simulink model "PropuestaControl"  (R2022b)
settings: Solver=ode4  StartTime=0.0  StopTime=60  FixedStep=0.001  RelTol=1e-3
values from neighbouring files (symbols this model uses):
  Ap = Am(:,1:20)    [IniciadorParametros.m]
  B = [zeros(n,n);eye(n,n)]    [IniciadorParametros.m]
  Psi1 = [V1 zeros(n,n)]    [IniciadorParametros.m]
  Psi2 = [zeros(n,n) V2]    [IniciadorParametros.m]
  V0 = Data(:,1)    [IniciadorParametros.m]
undefined symbols (not defined in the file or in its folder): A, P, W1, W2
settings Model: Creator=raul  LastModifiedBy=raul

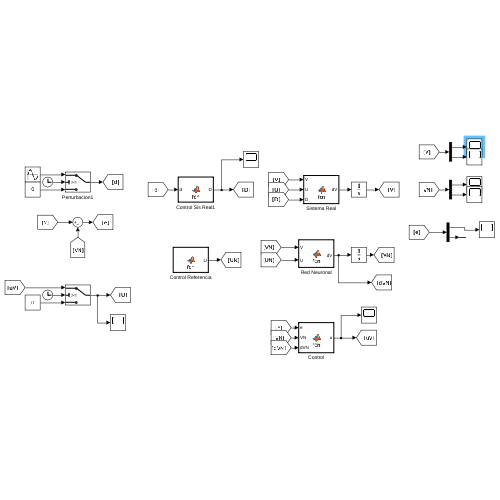
[thumbnail: Simulink's stored preview of the top-level diagram]
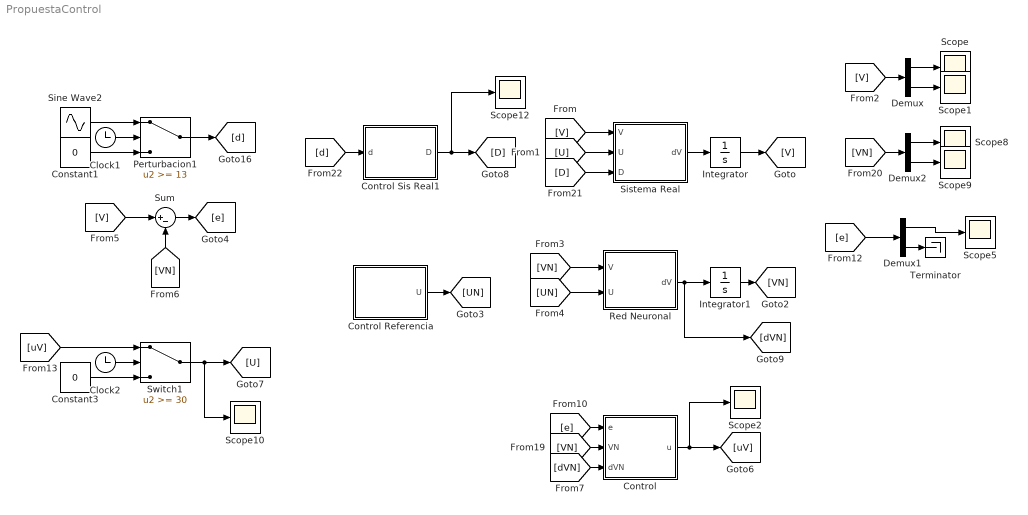
== system PropuestaControl ==
  Clock1 : Clock
  Clock2 : Clock
  Constant1 : Constant  Value=0
  Constant3 : Constant  Value=0
  Control : MATLAB Function  TreatAsAtomicUnit=on
  Control Referencia : MATLAB Function  TreatAsAtomicUnit=on
  Control Sis Real1 : MATLAB Function  TreatAsAtomicUnit=on
  Demux : Demux  Outputs=2
  Demux1 : Demux  Outputs=2
  Demux2 : Demux  Outputs=2
  Integrator : Integrator  InitialCondition=V0
  Integrator1 : Integrator  InitialCondition=V0
  Perturbacion1 : Switch  Threshold=13  SaturateOnIntegerOverflow=off  InputSameDT=off
  Red Neuronal : MATLAB Function  TreatAsAtomicUnit=on
  Scope{,1..2,5,8..10,12} (8 alike) : Scope
  Sine Wave2 : Sin  Frequency=5  SampleTime=0
  Sistema Real : MATLAB Function  TreatAsAtomicUnit=on
  Sum : Sum  Inputs=|+-
  Switch1 : Switch  Threshold=30  SaturateOnIntegerOverflow=off  InputSameDT=off
  Terminator : Terminator
  wires:
  Sistema Real/1(dV) -> Integrator/1
  Integrator/1 -> [V]
  [V] -> Sistema Real/1(V)
  [U] -> Sistema Real/2(U)
  [V] -> Demux/1
  Demux/1 -> Scope/1
  Demux/2 -> Scope1/1
  [VN] -> Red Neuronal/1(V)
  Red Neuronal/1(dV) -> [dVN], Integrator1/1
  Integrator1/1 -> [VN]
  [V] -> Sum/1
  [VN] -> Sum/2
  Perturbacion1/1 -> [d]
  Sine Wave2/1 -> Perturbacion1/1
  Clock1/1 -> Perturbacion1/2
  Constant1/1 -> Perturbacion1/3
  [UN] -> Red Neuronal/2(U)
  Control Referencia/1(U) -> [UN]
  Sum/1 -> [e]
  [e] -> Control/1(e)
  Control/1(u) -> Scope2/1, [uV]
  Switch1/1 -> Scope10/1, [U]
  Constant3/1 -> Switch1/3
  Clock2/1 -> Switch1/2
  [e] -> Demux1/1
  Demux1/1 -> Scope5/1
  Demux1/2 -> Terminator/1
  [VN] -> Control/2(VN)
  Demux2/1 -> Scope8/1
  Demux2/2 -> Scope9/1
  [VN] -> Demux2/1
  [uV] -> Switch1/1
  Control Sis Real1/1(D) -> Scope12/1, [D]
  [d] -> Control Sis Real1/1(d)
  [D] -> Sistema Real/3(D)
  [dVN] -> Control/3(dVN)

== matlab function PropuestaControl/Sistema Real ==
  data: V input; U input; dV output; W1 parameter; W2 parameter; Psi1 parameter; Psi2 parameter; B parameter; A parameter; D input
function dV  = fcn(V, U, W1, W2, Psi1, Psi2, B, A,D)

dV=A*V+B*(W1*sigmoid(Psi1,V)+W2*phi_sigmoid(Psi2,V)*U+W2*phi_sigmoid(Psi2,V)*D);


function s = sigmoid(b,x)
   s = 1./(1+exp(-b*x)); 
end



function phi = phi_sigmoid(bp, xp)
    % Comprueba que b y x tengan las dimensiones adecuadas
    [rows_b, cols_b] = size(bp);
%     [rows_x, cols_x] = size(xp);

    % Inicializa la matriz de salida
    phi = zeros(rows_b, rows_b); % Matriz de 20x20

    % Calcula la sigmoide combinando cada fila de b con el vector x
    for i = 1:rows_b
        phi(i, :) = 1 ./ (1 + exp(-bp(i, :) * xp)); % Producto y sigmoide
    end
end



end

== matlab function PropuestaControl/Red Neuronal ==
  data: V input; U input; dV output; W1 parameter; W2 parameter; Psi1 parameter; Psi2 parameter; B parameter; A parameter
function dV  = fcn(V, U, W1, W2, Psi1, Psi2, B, A)

dV=A*V+B*(W1*sigmoid(Psi1,V)+W2*phi_sigmoid(Psi2,V)*U);


function s = sigmoid(b,x)
   s = 1./(1+exp(-b*x)); 
end



function phi = phi_sigmoid(bp, xp)
    % Comprueba que b y x tengan las dimensiones adecuadas
    [rows_b, cols_b] = size(bp);
%     [rows_x, cols_x] = size(xp);

    % Inicializa la matriz de salida
    phi = zeros(rows_b, rows_b); % Matriz de 20x20

    % Calcula la sigmoide combinando cada fila de b con el vector x
    for i = 1:rows_b
        phi(i, :) = 1 ./ (1 + exp(-bp(i, :) * xp)); % Producto y sigmoide
    end
end



end

== matlab function PropuestaControl/Control Referencia ==
  data: U output
function U = fcn()%add Bw,w

U=zeros(20,1);

== matlab function PropuestaControl/Control ==
  data: u output; e input; Ap parameter; P parameter; W2 parameter; Psi2 parameter; VN input; dVN input; W1 parameter; Psi1 parameter
function u = fcn(e,Ap,P,W2,Psi2,VN,dVN, W1, Psi1)

x_star=dVN(1:20);
er=e(21:40);
k=10;



u1=pinv(W2*phi_sigmoid(Psi2,VN))*(x_star-Ap*VN(1:20)-W1*sigmoid(Psi1,VN));
u2=-k*P\sign(er);

u=u1+pinv(W2*phi_sigmoid(Psi2,VN))*u2;
% u=pinv(W2*phi_sigmoid(Psi2,VN))*u2;

function s = sigmoid(b,x)
   s = 1./(1+exp(-b*x)); 
end

function phi = phi_sigmoid(bp, xp)
    % Comprueba que b y x tengan las dimensiones adecuadas
    [rows_b, cols_b] = size(bp);
%     [rows_x, cols_x] = size(xp);

    % Inicializa la matriz de salida
    phi = zeros(rows_b, rows_b); % Matriz de 20x20

    % Calcula la sigmoide combinando cada fila de b con el vector x
    for i = 1:rows_b
        phi(i, :) = 1 ./ (1 + exp(-bp(i, :) * xp)); % Producto y sigmoide
    end
end

end

== matlab function PropuestaControl/Control Sis Real1 ==
  data: D output; d input; nodeDisturbe parameter
function D = fcn(d, nodeDisturbe)%add Bw,w

D=zeros(20,1);
D(nodeDisturbe,1)=d;
